simulink model "teste"  (R2021a)
settings: Solver=FixedStepAuto  StartTime=0.0  StopTime=500  FixedStep=10/100  RelTol=1e-3
settings Model: Creator=phcs  LastModifiedBy=phcs

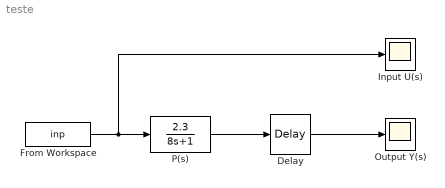
== system teste ==
  Delay : TransportDelay
  From Workspace : FromWorkspace  VariableName=inp
  Input U(s) : Scope
  Output Y(s) : Scope
  P(s) : TransferFcn  Numerator=[2.3]  Denominator=[8 1]  ContinuousStateAttributes="\"\""
  wires:
  Delay/1 -> Output Y(s)/1
  P(s)/1 -> Delay/1
  From Workspace/1 -> Input U(s)/1, P(s)/1
